simulink library "Linkage_Bumpstop_PtcldSurface"  (R2023a)
settings: Solver=ode23t  StartTime=0.0  StopTime=10.0  RelTol=1e-3
undefined symbols (not defined in the file): bumpstop_height, X, Y, Z
libraries: sm_lib x7
Description:
  | Component of Simscape Vehicle Templates Library
  | 
  | Copyright 2018-2024 The MathWorks, Inc.
settings Model: Creator=smiller  LastModifiedBy=smiller
settings SolverCC: AlgebraicLoopSolver=TrustRegion
settings DataIOCC: ReturnWorkspaceOutputs=off
settings DebuggingCC: UnconnectedInputMsg=warning  UnconnectedOutputMsg=warning  UnconnectedLineMsg=warning  ArithmeticOperatorsInVariantConditions=warning
settings ModelReferenceCC: EnableRefExpFcnMdlSchedulingChecks=on
settings SFSimCC: CustomCodeUndefinedFunction=UseInterfaceOnly

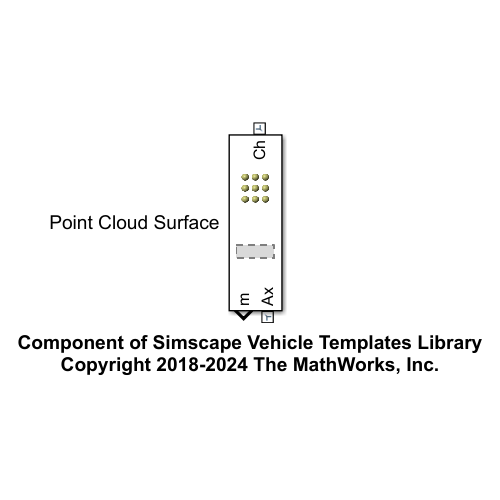
[thumbnail: Simulink's stored preview of the top-level diagram]
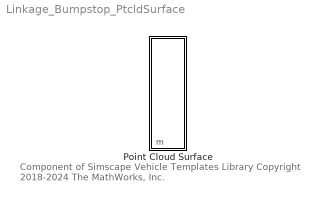
== system Linkage_Bumpstop_PtcldSurface ==
  note: Component of Simscape Vehicle Templates Library
      | Copyright 2018-2024 The MathWorks, Inc.
  Point Cloud Surface : Subsystem  mask{hp_bumpstop_body=0, hp_bumpstop_axle=0, bumpstop_ptcld=0, bumpstop_k=0, bumpstop_d=0, bumpstop_xTrans=0}
      mask prompts: hp_bumpstop_body "HP Bumpstop Chassis [xyz] (m)"; hp_bumpstop_axle "HP Bumpstop Axle [xyz] (m)"; bumpstop_ptcld "Point Cloud [xyz] (3 x npts) (m)"; bumpstop_k "Stiffness (N/m)"; bumpstop_d "Damping (N/(m/s))"; bumpstop_xTrans "Transition Depth (m)"
      mask Display: image('sm_car_bumpstop_ext_ptcldSurface.png')

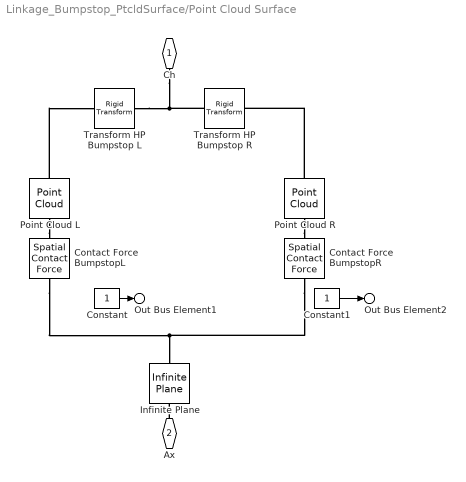
== system Linkage_Bumpstop_PtcldSurface/Point Cloud Surface ==
  Constant : Constant
  Constant1 : Constant
  Contact Force BumpstopL : sm_lib/Forces and Torques/Spatial Contact Force  SenseContactBaseRotation=off  SenseContactBaseTranslation=off  CoefficientOfDynamicFriction=0.3  CoefficientOfStaticFriction=0.5  NormalDamping=bumpstop_d  NormalDampingUnits=N/(m/s)  SenseContactSignal=off  NormalStiffness=bumpstop_k  NormalStiffnessUnits=N/m  FrictionalCriticalVelocity=1e-3  FrictionalCriticalVelocityUnits=m/s  ZeroCrossDetectContactStartAndEnd=off  SenseContactFollowerRotation=off  SenseContactFollowerTranslation=off  FrictionType=None  SenseFrictionalForceMagnitude=off  SenseNormalForceMagnitude=off  NormalForceType=SmoothSpringDamper  SenseNormalVelocity=off  SenseSeparationDistance=off  SenseTangentialVelocity=off  NormalTransitionRegionWidth=bumpstop_xTrans  NormalTransitionRegionWidthUnits=m
  Contact Force BumpstopR : sm_lib/Forces and Torques/Spatial Contact Force  SenseContactBaseRotation=off  SenseContactBaseTranslation=off  CoefficientOfDynamicFriction=0.3  CoefficientOfStaticFriction=0.5  NormalDamping=bumpstop_d  NormalDampingUnits=N/(m/s)  SenseContactSignal=off  NormalStiffness=bumpstop_k  NormalStiffnessUnits=N/m  FrictionalCriticalVelocity=1e-3  FrictionalCriticalVelocityUnits=m/s  ZeroCrossDetectContactStartAndEnd=off  SenseContactFollowerRotation=off  SenseContactFollowerTranslation=off  FrictionType=None  SenseFrictionalForceMagnitude=off  SenseNormalForceMagnitude=off  NormalForceType=SmoothSpringDamper  SenseNormalVelocity=off  SenseSeparationDistance=off  SenseTangentialVelocity=off  NormalTransitionRegionWidth=bumpstop_xTrans  NormalTransitionRegionWidthUnits=m
  Infinite Plane : sm_lib/Curves and Surfaces/Infinite Plane  GraphicType=Rectangle  GraphicPlaneWidth=bumpstop_height*3  GraphicPlaneWidthUnits=m  GraphicPlaneHeight=(hp_bumpstop_body(2)+bumpstop_height)*2  GraphicPlaneHeightUnits=m  GraphicVisPropType=SimpleVisualProperties  GraphicDiffuseColor=[0.5 0.5 0.5]  GraphicOpacity=0.25  GraphicSpecularColor=[0.5 0.5 0.5 1.0]  GraphicAmbientColor=[0.15 0.15 0.15 1.0]  GraphicEmissiveColor=[0.0 0.0 0.0 1.0]  GraphicShininess=75
  Point Cloud L : sm_lib/Curves and Surfaces/Point Cloud  CoordinatesMatrix=bumpstop_ptcld  CoordinatesMatrixUnits=m  GraphicType=MarkerCloud  GraphicSphereRadius=Visual.Shock.bumpstop.ptRad  GraphicSphereRadiusUnits=m  GraphicVisPropType=SimpleVisualProperties  GraphicDiffuseColor=Visual.Bumpstop.clr  GraphicOpacity=Visual.part.opc  GraphicSpecularColor=[0.5 0.5 0.5 1.0]  GraphicAmbientColor=[0.15 0.15 0.15 1.0]  GraphicEmissiveColor=[0.0 0.0 0.0 1.0]  GraphicShininess=75
  Point Cloud R : sm_lib/Curves and Surfaces/Point Cloud  CoordinatesMatrix=bumpstop_ptcld.*[1 -1 1]  CoordinatesMatrixUnits=m  GraphicType=MarkerCloud  GraphicSphereRadius=Visual.Shock.bumpstop.ptRad  GraphicSphereRadiusUnits=m  GraphicVisPropType=SimpleVisualProperties  GraphicDiffuseColor=Visual.Bumpstop.clr  GraphicOpacity=Visual.part.opc  GraphicSpecularColor=[0.5 0.5 0.5 1.0]  GraphicAmbientColor=[0.15 0.15 0.15 1.0]  GraphicEmissiveColor=[0.0 0.0 0.0 1.0]  GraphicShininess=75
  Transform HP Bumpstop L : sm_lib/Frames and Transforms/Rigid Transform  TranslationMethod=Cartesian  TranslationStandardOffset=0  TranslationStandardOffsetUnits=m  TranslationStandardAxis=+Z  TranslationCartesianOffset=hp_bumpstop_body  TranslationCartesianOffsetUnits=m  TranslationROffset=0  TranslationROffsetUnits=m  TranslationZOffset=0  TranslationZOffsetUnits=m  TranslationThetaOffset=0  TranslationThetaOffsetUnits=deg  RotationMethod=None  RotationAngleUnits=deg  RotationStandardAxis=+Z  RotationAngle=0  RotationArbitraryAxis=[0 0 1]  FollAlignAxisA=+X  BaseAlignAxisA=+Y  FollAlignAxisB=+Y  BaseAlignAxisB=+Z  RotationSequenceAxes=FollowerAxes  RotationSequence=XYX  RotationSequenceAngles=[0 0 0]  RotationSequenceAnglesUnits=deg  RotationMatrix=[1 0 0;0 1 0;0 0 1]  Quaternion=[1 0 0 0]
  Transform HP Bumpstop R : sm_lib/Frames and Transforms/Rigid Transform  TranslationMethod=Cartesian  TranslationStandardOffset=0  TranslationStandardOffsetUnits=m  TranslationStandardAxis=+Z  TranslationCartesianOffset=hp_bumpstop_body.*[1 -1 1]  TranslationCartesianOffsetUnits=m  TranslationROffset=0  TranslationROffsetUnits=m  TranslationZOffset=0  TranslationZOffsetUnits=m  TranslationThetaOffset=0  TranslationThetaOffsetUnits=deg  RotationMethod=None  RotationAngleUnits=deg  RotationStandardAxis=+Z  RotationAngle=0  RotationArbitraryAxis=[0 0 1]  FollAlignAxisA=+X  BaseAlignAxisA=+Y  FollAlignAxisB=+Y  BaseAlignAxisB=+Z  RotationSequenceAxes=FollowerAxes  RotationSequence=XYX  RotationSequenceAngles=[0 0 0]  RotationSequenceAnglesUnits=deg  RotationMatrix=[1 0 0;0 1 0;0 0 1]  Quaternion=[1 0 0 0]
  Ch : PMIOPort  Side=Left
  Ax : PMIOPort  Port=2  Side=Right
  Out Bus Element1 : Outport  PortName=m  Element=fnL
  Out Bus Element2 : Outport  PortName=m  Element=fnR
  wires:
  Constant1/1 -> Out Bus Element2/1
  Constant/1 -> Out Bus Element1/1
  connections:
  Point Cloud R/LConn1 -- Transform HP Bumpstop R/RConn1
  Contact Force BumpstopL/RConn1 -- Contact Force BumpstopR/RConn1 -- Infinite Plane/RConn1
  Point Cloud R/RConn1 -- Contact Force BumpstopR/LConn1
  Point Cloud L/RConn1 -- Contact Force BumpstopL/LConn1
  Point Cloud L/LConn1 -- Transform HP Bumpstop L/RConn1
  Ax/RConn1 -- Infinite Plane/LConn1
  Transform HP Bumpstop R/LConn1 -- Transform HP Bumpstop L/LConn1 -- Ch/RConn1
